simulink library "MCHP_Blockset"  (Simulink 7.5)
(part 3 of 9)

      mask prompts: ACLKCON "Enable fast conversion using Auxiliary clock"; ADC_FRACT "Conversion Format (common to all ADC blocks)"; ADC_NRE "Noise Reduction Enabled (might add delays)"; DMA_Size "Multiple trigger - Vector output - for ADC[0-6] of current block"; ADC_Synchronisation "ADC Sample and Conversion"; ADC_Trig "User defined trigger:"; ADC_TrigTimeStep "Synchronisation with model Time Step:"; ADC_TrigInfo "ADC Trigger Info"; SampleTime "Block output sample time"; ADC_Info "Infos"; ADC0_pin "Analog input pin"; ADC0_R "Input Impedance"; ADC0_res "Resolution of conversion"; ADC0_signed "Output format"; ADC0_FILTER "Filter / Oversampling"; ADC0_FILTER_nSamples "Filter / Oversampling burst of:"; ADC0_STRGEN "Initial trigger option:"; ADC0_STRGEN_on "Initial trigger option:"; ADC0_SSAMPEN "Ensure synchronous sampling (might add a delay)"; ADC0_Info "ADC0 Info"; ADC1_pin "Analog input pin"; ADC1_pin_TXT "ADC0_pin_TXT"; ADC1_R "Input Impedance"; ADC1_res "Resolution of conversion"; ADC1_signed "Output format"; ADC1_FILTER "Filter / Oversampling"; ADC1_FILTER_nSamples "Filter / Oversampling burst of:"; ADC1_STRGEN "Initial trigger option:"; ADC1_STRGEN_on "Initial trigger option:"; ADC1_SSAMPEN "Ensure synchronous sampling (might add a delay)"; ADC1_Info "ADC1 Infos"; ADC2_pin "Analog input pin"; ADC2_R "Input Impedance"; ADC2_res "Resolution of conversion"; ADC2_signed "Output format"; ADC2_FILTER "Filter / Oversampling"; ADC2_FILTER_nSamples "Filter / Oversampling burst of:"; ADC2_STRGEN "Initial trigger option:"; ADC2_STRGEN_on "Initial trigger option:"; ADC2_SSAMPEN "Ensure synchronous sampling (might add a delay)"; ADC2_Info "ADC2 Infos"; ADC3_pin "Analog input pin"; ADC3_R "Input Impedance"; ADC3_res "Resolution of conversion"; ADC3_signed "Output format"; ADC3_FILTER "Filter / Oversampling"; ADC3_FILTER_nSamples "Filter / Oversampling burst of:"; ADC3_STRGEN "Initial trigger option:"; ADC3_STRGEN_on "Initial trigger option:"; ADC3_SSAMPEN "Ensure synchronous sampling (might add a delay)"; ADC3_Info "ADC3 Infos"; ADC4_pin "Analog input pin"; ADC4_R "Input Impedance"; ADC4_res "Resolution of conversion"; ADC4_signed "Output format"; ADC4_FILTER "Filter / Oversampling"; ADC4_FILTER_nSamples "Filter / Oversampling burst of:"; ADC4_STRGEN "Initial trigger option:"; ADC4_STRGEN_on "Initial trigger option:"; ADC4_SSAMPEN "Ensure synchronous sampling (might add a delay)"; ADC4_Info "ADC4 Infos"; ADC5_pin "Analog input pin"; ADC5_R "Input Impedance"; ADC5_res "Resolution of conversion"; ADC5_signed "Output format"; ADC5_FILTER "Filter / Oversampling"; ADC5_FILTER_nSamples "Filter / Oversampling burst of:"; ADC5_STRGEN "Initial trigger option:"; ADC5_STRGEN_on "Initial trigger option:"; ADC5_SSAMPEN "Ensure synchronous sampling (might add a delay)"; ADC5_Info "ADC5 Infos"; ADC6_pin "Analog input pin"; ADC6_R "Input Impedance"; ADC6_res "Resolution of conversion"; ADC6_signed "Output format"; ADC6_FILTER "Filter / Oversampling"; ADC6_FILTER_nSamples "Filter / Oversampling burst of:"; ADC6_STRGEN "Initial trigger option:"; ADC6_STRGEN_on "Initial trigger option:"; ADC6_SSAMPEN "Ensure synchronous sampling (might add a delay)"; ADC6_Info "ADC6 Infos"; ADC7_R "ADC7 Input Impedance (Class 2 and 3 inputs)"; ADC7_res "ADC7 Resolution of conversion (Class 2 and 3 inputs)"; ADC7_AN0 "AN0 pin"; ADC7_AN1 "AN1 pin"; ADC7_AN2 "AN2_pin"; ADC7_AN3 "AN3_pin"; ADC7_AN4 ""; ADC7_AN5 ""; ADC7_AN6 "AN6 / B1 / Pin[32]"; ADC7_AN7 "AN7 / B2 / Pin[33]"; ADC7_AN8 "AN8 / C1 / Pin[31]"; ADC7_AN9 "AN9 / C2 / Pin[36]"; ADC7_AN10 "AN10 / C10 / Pin[28]"; ADC7_AN11 "AN11 / C9 / Pin[27]"; ADC7_AN12 "AN12 / C11 / Pin[19]"; ADC7_AN13 ""; ADC7_AN14 "AN14 / C12 / Pin[20]"; ADC7_AN15 ""; ADC7_AN16 ""; ADC7_AN17 "AN17 / C6 / Pin[4]"; ADC7_AN18 "AN18 / B3 / Pin[34]"; ADC7_AN19 "AN19 / B5 / Pin[43]"; ADC7_AN20 "AN20 / B6 / Pin[44]"; ADC7_AN21 "AN21 / B7 / Pin[1]"; ADC7_AN22 ""; ADC7_AN23 ""; ADC7_AN24 ""; ADC7_AN25 ""; ADC7_AN26 ""; ADC7_AN27 ""; ADC7_AN28 ""; ADC7_AN29 ""; ADC7_AN30 ""; ADC7_AN31 ""; IVref "Vref (1.2V)"; IVTemp "Temp"; ADC7_Info "Shared ADC Infos"
      mask init:
      | MCHP_ADC_HighSpeed_SAR_dsPIC_Callback(gcbh,'INITIALISATION');
      settings: CopyFcn=MCHP_ADC_HighSpeed_SAR_dsPIC_Callback(gcbh,'CopyFcn');  PreSaveFcn=MCHP_Fun.PreSaveFcn_DynamicOptions(gcbh);  OpenFcn=MCHP_ADC_HighSpeed_SAR_dsPIC_Callback(gcbh,'OPEN');
      mask StyleString: popup(Not used|Optimized for PWM resolution & ADC conversion speed|Optimized for PWM accuracy),popup(Integer (right aligned)|Fractional (left aligned)),checkbox,popup(Single trigger - (default)|1 trig / 1 element output (ping pong buffer)|2 trig / 2 elements output (ping-pong buffer)|3 trig / 3 elements output (ping-pong buffer)|4 trig / 4 elements output (ping-pong buffer)),popup(Triggered at end of previous time step|Triggered by custom source|Continuously triggered. Output is last conversion),popup(Dynamic Options),edit,popup(None (independant)|Trig model step after all sample using this trigger are converted|Trig model step after all sample from this block are converted),edit,edit,edit,edit,edit,edit,edit,edit,edit,edit,edit,edit,popup(Dynamic Options),edit,popup(< 200 Ohm|< 500 Ohm|< 1    kOhm|< 2    kOhm|< 5    kOhm|< 10   kOhm|< 20   kOhm|< 50   kOhm|< 100  kOhm|< 200  kOhm|< 500  kOhm|max sampling time),popup(12 bits|10 bits|8 bits|6 bits),popup(unsigned 16 bits|signed 16 bits),popup(No Oversampling|Burst convert of n samples are Summed|Burst convert of n samples are Averaged),popup(2 samples|4 samples|8 samples|16 samples|32 samples|64 samples|128 samples|256 samples),popup(End sampling and start conversion|Start sampling followed by conversion),popup(Start sampling followed by conversion),checkbox,edit,popup(Dynamic Options),edit,popup(< 200 Ohm|< 500 Ohm|< 1    kOhm|< 2    kOhm|< 5    kOhm|< 10   kOhm|< 20   kOhm|< 50   kOhm|< 100  kOhm|< 200  kOhm|< 500  kOhm|max sampling time),popup(12 bits|10 bits|8 bits|6 bits),popup(unsigned 16 bits|signed 16 bits),popup(No Oversampling|Burst convert of n samples are Summed|Burst convert of n samples are Averaged),popup(2 samples|4 samples|8 samples|16 samples|32 samples|64 samples|128 samples|256 samples),popup(End sampling and start conversion|Start sampling followed by conversion),popup(Start sampling followed by conversion),checkbox,edit,popup(Dynamic Options),edit,popup(< 200 Ohm|< 500 Ohm|< 1    kOhm|< 2    kOhm|< 5    kOhm|< 10   kOhm|< 20   kOhm|< 50   kOhm|< 100  kOhm|< 200  kOhm|< 500  kOhm|max sampling time),popup(12 bits|10 bits|8 bits|6 bits),popup(unsigned 16 bits|signed 16 bits),popup(No Oversampling|Burst convert of n samples are Summed|Burst convert of n samples are Averaged),popup(2 samples|4 samples|8 samples|16 samples|32 samples|64 samples|128 samples|256 samples),popup(End sampling and start conversion|Start sampling followed by conversion),popup(Start sampling followed by conversion),checkbox,edit,popup(Dynamic Options),edit,popup(< 200 Ohm|< 500 Ohm|< 1    kOhm|< 2    kOhm|< 5    kOhm|< 10   kOhm|< 20   kOhm|< 50   kOhm|< 100  kOhm|< 200  kOhm|< 500  kOhm|max sampling time),popup(12 bits|10 bits|8 bits|6 bits),popup(unsigned 16 bits|signed 16 bits),popup(No Oversampling|Burst convert of n samples are Summed|Burst convert of n samples are Averaged),popup(2 samples|4 samples|8 samples|16 samples|32 samples|64 samples|128 samples|256 samples),popup(End sampling and start conversion|Start sampling followed by conversion),popup(Start sampling followed by conversion),checkbox,edit,popup(Dynamic Options),edit,popup(< 200 Ohm|< 500 Ohm|< 1    kOhm|< 2    kOhm|< 5    kOhm|< 10   kOhm|< 20   kOhm|< 50   kOhm|< 100  kOhm|< 200  kOhm|< 500  kOhm|max sampling time),popup(12 bits|10 bits|8 bits|6 bits),popup(unsigned 16 bits|signed 16 bits),popup(No Oversampling|Burst convert of n samples are Summed|Burst convert of n samples are Averaged),popup(2 samples|4 samples|8 samples|16 samples|32 samples|64 samples|128 samples|256 samples),popup(End sampling and start conversion|Start sampling followed by conversion),popup(Start sampling followed by conversion),checkbox,edit,popup(Dynamic Options),edit,popup(< 200 Ohm|< 500 Ohm|< 1    kOhm|< 2    kOhm|< 5    kOhm|< 10   kOhm|< 20   kOhm|< 50   kOhm|< 100  kOhm|< 200  kOhm|< 500  kOhm|max sampling time),popup(12 bits|10 bits|8 bits|6 bits),popup(unsigned 16 bits|signed 16 bits),popup(No Oversampling|Burst convert of n samples are Summed|Burst convert of n samples are Averaged),popup(2 samples|4 samples|8 samples|16 samples|32 samples|64 samples|128 samples|256 samples),popup(End sampling and start conversion|Start sampling followed by conversion),popup(Start sampling followed by conversion),checkbox,edit,popup(Dynamic Options),edit,popup(< 200 Ohm|< 500 Ohm|< 1    kOhm|< 2    kOhm|< 5    kOhm|< 10   kOhm|< 20   kOhm|< 50   kOhm|< 100  kOhm|< 200  kOhm|< 500  kOhm|max sampling time),popup(12 bits|10 bits|8 bits|6 bits),popup(unsigned 16 bits|signed 16 bits),popup(No Oversampling|Burst convert of n samples are Summed|Burst convert of n samples are Averaged),popup(2 samples|4 samples|8 samples|16 samples|32 samples|64 samples|128 samples|256 samples),popup(End sampling and start conversion|Start sampling followed by conversion),popup(Start sampling followed by conversion),checkbox,edit,popup(< 200 Ohm|< 500 Ohm|< 1    kOhm|< 2    kOhm|< 5    kOhm|< 10   kOhm|< 20   kOhm|< 50   kOhm|< 100  kOhm|< 200  kOhm|< 500  kOhm|max sampling time),popup(12 bits|10 bits|8 bits|6 bits),popup(Not used|unsigned int16 |signed int16|---Burst Sample with internal Digital filter---|2 samples averaged - unsigned int16|4 samples averaged - unsigned int16|8 samples averaged - unsigned int16|16 samples averaged - unsigned int16|32 samples averaged - unsigned int16|64 samples averaged - unsigned int16|128 samples averaged - unsigned int16|256 samples averaged - unsigned int16|----|2 samples averaged - signed int16|4 samples averaged - signed int16|8 samples averaged - signed int16|16 samples averaged - signed int16|32 samples averaged - signed int16|64 samples averaged - signed int16|128 samples averaged - signed int16|256 samples averaged - signed int16|-----|4 samples summed - unsigned int16|8 samples summed - unsigned int16|16 samples summed - unsigned int16|32 samples summed - unsigned int16|64 samples summed - unsigned int16|128 samples summed - unsigned int16|256 samples summed - unsigned int16|------|2 samples summed - signed int16|4 samples summed - signed int16|8 samples summed - signed int16|16 samples summed - signed int16|32 samples summed - signed int16),popup(Not used|unsigned int16 |signed int16|---Burst Sample with internal Digital filter---|2 samples averaged - unsigned int16|4 samples averaged - unsigned int16|8 samples averaged - unsigned int16|16 samples averaged - unsigned int16|32 samples averaged - unsigned int16|64 samples averaged - unsigned int16|128 samples averaged - unsigned int16|256 samples averaged - unsigned int16|----|2 samples averaged - signed int16|4 samples averaged - signed int16|8 samples averaged - signed int16|16 samples averaged - signed int16|32 samples averaged - signed int16|64 samples averaged - signed int16|128 samples averaged - signed int16|256 samples averaged - signed int16|-----|4 samples summed - unsigned int16|8 samples summed - unsigned int16|16 samples summed - unsigned int16|32 samples summed - unsigned int16|64 samples summed - unsigned int16|128 samples summed - unsigned int16|256 samples summed - unsigned int16|------|2 samples summed - signed int16|4 samples summed - signed int16|8 samples summed - signed int16|16 samples summed - signed int16|32 samples summed - signed int16|64 samples summed - signed int16|128 samples summed - signed int16|256 samples summed - signed int16),popup(Not used|unsigned int16 |signed int16|---Burst Sample with internal Digital filter---|2 samples averaged - unsigned int16|4 samples averaged - unsigned int16|8 samples averaged - unsigned int16|16 samples averaged - unsigned int16|32 samples averaged - unsigned int16|64 samples averaged - unsigned int16|128 samples averaged - unsigned int16|256 samples averaged - unsigned int16|----|2 samples averaged - signed int16|4 samples averaged - signed int16|8 samples averaged - signed int16|16 samples averaged - signed int16|32 samples averaged - signed int16|64 samples averaged - signed int16|128 samples averaged - signed int16|256 samples averaged - signed int16|-----|4 samples summed - unsigned int16|8 samples summed - unsigned int16|16 samples summed - unsigned int16|32 samples summed - unsigned int16|64 samples summed - unsigned int16|128 samples summed - unsigned int16|256 samples summed - unsigned int16|------|2 samples summed - signed int16|4 samples summed - signed int16|8 samples summed - signed int16|16 samples summed - signed int16|32 samples summed - signed int16|64 samples summed - signed int16|128 samples summed - signed int16|256 samples summed - signed int16),popup(Not used|unsigned int16 |signed int16|---Burst Sample with internal Digital filter---|2 samples averaged - unsigned int16|4 samples averaged - unsigned int16|8 samples averaged - unsigned int16|16 samples averaged - unsigned int16|32 samples averaged - unsigned int16|64 samples averaged - unsigned int16|128 samples averaged - unsigned int16|256 samples averaged - unsigned int16|----|2 samples averaged - signed int16|4 samples averaged - signed int16|8 samples averaged - signed int16|16 samples averaged - signed int16|32 samples averaged - signed int16|64 samples averaged - signed int16|128 samples averaged - signed int16|256 samples averaged - signed int16|-----|4 samples summed - unsigned int16|8 samples summed - unsigned int16|16 samples summed - unsigned int16|32 samples summed - unsigned int16|64 samples summed - unsigned int16|128 samples summed - unsigned int16|256 samples summed - unsigned int16|------|2 samples summed - signed int16|4 samples summed - signed int16|8 samples summed - signed int16|16 samples summed - signed int16|32 samples summed - signed int16|64 samples summed - signed int16|128 samples summed - signed int16|256 samples summed - signed int16),popup(Not used|unsigned int16 |signed int16|---Burst Sample with internal Digital filter---|2 samples averaged - unsigned int16|4 samples averaged - unsigned int16|8 samples averaged - unsigned int16|16 samples averaged - unsigned int16|32 samples averaged - unsigned int16|64 samples averaged - unsigned int16|128 samples averaged - unsigned int16|256 samples averaged - unsigned int16|----|2 samples averaged - signed int16|4 samples averaged - signed int16|8 samples averaged - signed int16|16 samples averaged - signed int16|32 samples averaged - signed int16|64 samples averaged - signed int16|128 samples averaged - signed int16|256 samples averaged - signed int16|-----|4 samples summed - unsigned int16|8 samples summed - unsigned int16|16 samples summed - unsigned int16|32 samples summed - unsigned int16|64 samples summed - unsigned int16|128 samples summed - unsigned int16|256 samples summed - unsigned int16|------|2 samples summed - signed int16|4 samples summed - signed int16|8 samples summed - signed int16|16 samples summed - signed int16|32 samples summed - signed int16|64 samples summed - signed int16|128 samples summed - signed int16|256 samples summed - signed int16),popup(Not used|unsigned int16 |signed int16|---Burst Sample with internal Digital filter---|2 samples averaged - unsigned int16|4 samples averaged - unsigned int16|8 samples averaged - unsigned int16|16 samples averaged - unsigned int16|32 samples averaged - unsigned int16|64 samples averaged - unsigned int16|128 samples averaged - unsigned int16|256 samples averaged - unsigned int16|----|2 samples averaged - signed int16|4 samples averaged - signed int16|8 samples averaged - signed int16|16 samples averaged - signed int16|32 samples averaged - signed int16|64 samples averaged - signed int16|128 samples averaged - signed int16|256 samples averaged - signed int16|-----|4 samples summed - unsigned int16|8 samples summed - unsigned int16|16 samples summed - unsigned int16|32 samples summed - unsigned int16|64 samples summed - unsigned int16|128 samples summed - unsigned int16|256 samples summed - unsigned int16|------|2 samples summed - signed int16|4 samples summed - signed int16|8 samples summed - signed int16|16 samples summed - signed int16|32 samples summed - signed int16|64 samples summed - signed int16|128 samples summed - signed int16|256 samples summed - signed int16),popup(Not used|unsigned int16 |signed int16|---Burst Sample with internal Digital filter---|2 samples averaged - unsigned int16|4 samples averaged - unsigned int16|8 samples averaged - unsigned int16|16 samples averaged - unsigned int16|32 samples averaged - unsigned int16|64 samples averaged - unsigned int16|128 samples averaged - unsigned int16|256 samples averaged - unsigned int16|----|2 samples averaged - signed int16|4 samples averaged - signed int16|8 samples averaged - signed int16|16 samples averaged - signed int16|32 samples averaged - signed int16|64 samples averaged - signed int16|128 samples averaged - signed int16|256 samples averaged - signed int16|-----|4 samples summed - unsigned int16|8 samples summed - unsigned int16|16 samples summed - unsigned int16|32 samples summed - unsigned int16|64 samples summed - unsigned int16|128 samples summed - unsigned int16|256 samples summed - unsigned int16|------|2 samples summed - signed int16|4 samples summed - signed int16|8 samples summed - signed int16|16 samples summed - signed int16|32 samples summed - signed int16|64 samples summed - signed int16|128 samples summed - signed int16|256 samples summed - signed int16),popup(Not used|unsigned int16 |signed int16|---Burst Sample with internal Digital filter---|2 samples averaged - unsigned int16|4 samples averaged - unsigned int16|8 samples averaged - unsigned int16|16 samples averaged - unsigned int16|32 samples averaged - unsigned int16|64 samples averaged - unsigned int16|128 samples averaged - unsigned int16|256 samples averaged - unsigned int16|----|2 samples averaged - signed int16|4 samples averaged - signed int16|8 samples averaged - signed int16|16 samples averaged - signed int16|32 samples averaged - signed int16|64 samples averaged - signed int16|128 samples averaged - signed int16|256 samples averaged - signed int16|-----|4 samples summed - unsigned int16|8 samples summed - unsigned int16|16 samples summed - unsigned int16|32 samples summed - unsigned int16|64 samples summed - unsigned int16|128 samples summed - unsigned int16|256 samples summed - unsigned int16|------|2 samples summed - signed int16|4 samples summed - signed int16|8 samples summed - signed int16|16 samples summed - signed int16|32 samples summed - signed int16|64 samples summed - signed int16|128 samples summed - signed int16|256 samples summed - signed int16),popup(Not used|unsigned int16 |signed int16|---Burst Sample with internal Digital filter---|2 samples averaged - unsigned int16|4 samples averaged - unsigned int16|8 samples averaged - unsigned int16|16 samples averaged - unsigned int16|32 samples averaged - unsigned int16|64 samples averaged - unsigned int16|128 samples averaged - unsigned int16|256 samples averaged - unsigned int16|----|2 samples averaged - signed int16|4 samples averaged - signed int16|8 samples averaged - signed int16|16 samples averaged - signed int16|32 samples averaged - signed int16|64 samples averaged - signed int16|128 samples averaged - signed int16|256 samples averaged - signed int16|-----|4 samples summed - unsigned int16|8 samples summed - unsigned int16|16 samples summed - unsigned int16|32 samples summed - unsigned int16|64 samples summed - unsigned int16|128 samples summed - unsigned int16|256 samples summed - unsigned int16|------|2 samples summed - signed int16|4 samples summed - signed int16|8 samples summed - signed int16|16 samples summed - signed int16|32 samples summed - signed int16|64 samples summed - signed int16|128 samples summed - signed int16|256 samples summed - signed int16),popup(Not used|unsigned int16 |signed int16|---Burst Sample with internal Digital filter---|2 samples averaged - unsigned int16|4 samples averaged - unsigned int16|8 samples averaged - unsigned int16|16 samples averaged - unsigned int16|32 samples averaged - unsigned int16|64 samples averaged - unsigned int16|128 samples averaged - unsigned int16|256 samples averaged - unsigned int16|----|2 samples averaged - signed int16|4 samples averaged - signed int16|8 samples averaged - signed int16|16 samples averaged - signed int16|32 samples averaged - signed int16|64 samples averaged - signed int16|128 samples averaged - signed int16|256 samples averaged - signed int16|-----|4 samples summed - unsigned int16|8 samples summed - unsigned int16|16 samples summed - unsigned int16|32 samples summed - unsigned int16|64 samples summed - unsigned int16|128 samples summed - unsigned int16|256 samples summed - unsigned int16|------|2 samples summed - signed int16|4 samples summed - signed int16|8 samples summed - signed int16|16 samples summed - signed int16|32 samples summed - signed int16|64 samples summed - signed int16|128 samples summed - signed int16|256 samples summed - signed int16),popup(Not used|unsigned int16 |signed int16|---Burst Sample with internal Digital filter---|2 samples averaged - unsigned int16|4 samples averaged - unsigned int16|8 samples averaged - unsigned int16|16 samples averaged - unsigned int16|32 samples averaged - unsigned int16|64 samples averaged - unsigned int16|128 samples averaged - unsigned int16|256 samples averaged - unsigned int16|----|2 samples averaged - signed int16|4 samples averaged - signed int16|8 samples averaged - signed int16|16 samples averaged - signed int16|32 samples averaged - signed int16|64 samples averaged - signed int16|128 samples averaged - signed int16|256 samples averaged - signed int16|-----|4 samples summed - unsigned int16|8 samples summed - unsigned int16|16 samples summed - unsigned int16|32 samples summed - unsigned int16|64 samples summed - unsigned int16|128 samples summed - unsigned int16|256 samples summed - unsigned int16|------|2 samples summed - signed int16|4 samples summed - signed int16|8 samples summed - signed int16|16 samples summed - signed int16|32 samples summed - signed int16|64 samples summed - signed int16|128 samples summed - signed int16|256 samples summed - signed int16),popup(Not used|unsigned int16 |signed int16|---Burst Sample with internal Digital filter---|2 samples averaged - unsigned int16|4 samples averaged - unsigned int16|8 samples averaged - unsigned int16|16 samples averaged - unsigned int16|32 samples averaged - unsigned int16|64 samples averaged - unsigned int16|128 samples averaged - unsigned int16|256 samples averaged - unsigned int16|----|2 samples averaged - signed int16|4 samples averaged - signed int16|8 samples averaged - signed int16|16 samples averaged - signed int16|32 samples averaged - signed int16|64 samples averaged - signed int16|128 samples averaged - signed int16|256 samples averaged - signed int16|-----|4 samples summed - unsigned int16|8 samples summed - unsigned int16|16 samples summed - unsigned int16|32 samples summed - unsigned int16|64 samples summed - unsigned int16|128 samples summed - unsigned int16|256 samples summed - unsigned int16|------|2 samples summed - signed int16|4 samples summed - signed int16|8 samples summed - signed int16|16 samples summed - signed int16|32 samples summed - signed int16|64 samples summed - signed int16|128 samples summed - signed int16|256 samples summed - signed int16),popup(Not used|unsigned int16 |signed int16|---Burst Sample with internal Digital filter---|2 samples averaged - unsigned int16|4 samples averaged - unsigned int16|8 samples averaged - unsigned int16|16 samples averaged - unsigned int16|32 samples averaged - unsigned int16|64 samples averaged - unsigned int16|128 samples averaged - unsigned int16|256 samples averaged - unsigned int16|----|2 samples averaged - signed int16|4 samples averaged - signed int16|8 samples averaged - signed int16|16 samples averaged - signed int16|32 samples averaged - signed int16|64 samples averaged - signed int16|128 samples averaged - signed int16|256 samples averaged - signed int16|-----|4 samples summed - unsigned int16|8 samples summed - unsigned int16|16 samples summed - unsigned int16|32 samples summed - unsigned int16|64 samples summed - unsigned int16|128 samples summed - unsigned int16|256 samples summed - unsigned int16|------|2 samples summed - signed int16|4 samples summed - signed int16|8 samples summed - signed int16|16 samples summed - signed int16|32 samples summed - signed int16|64 samples summed - signed int16|128 samples summed - signed int16|256 samples summed - signed int16),popup(Not used|unsigned int16 |signed int16|---Burst Sample with internal Digital filter---|2 samples averaged - unsigned int16|4 samples averaged - unsigned int16|8 samples averaged - unsigned int16|16 samples averaged - unsigned int16|32 samples averaged - unsigned int16|64 samples averaged - unsigned int16|128 samples averaged - unsigned int16|256 samples averaged - unsigned int16|----|2 samples averaged - signed int16|4 samples averaged - signed int16|8 samples averaged - signed int16|16 samples averaged - signed int16|32 samples averaged - signed int16|64 samples averaged - signed int16|128 samples averaged - signed int16|256 samples averaged - signed int16|-----|4 samples summed - unsigned int16|8 samples summed - unsigned int16|16 samples summed - unsigned int16|32 samples summed - unsigned int16|64 samples summed - unsigned int16|128 samples summed - unsigned int16|256 samples summed - unsigned int16|------|2 samples summed - signed int16|4 samples summed - signed int16|8 samples summed - signed int16|16 samples summed - signed int16|32 samples summed - signed int16|64 samples summed - signed int16|128 samples summed - signed int16|256 samples summed - signed int16),popup(Not used|unsigned int16 |signed int16|---Burst Sample with internal Digital filter---|2 samples averaged - unsigned int16|4 samples averaged - unsigned int16|8 samples averaged - unsigned int16|16 samples averaged - unsigned int16|32 samples averaged - unsigned int16|64 samples averaged - unsigned int16|128 samples averaged - unsigned int16|256 samples averaged - unsigned int16|----|2 samples averaged - signed int16|4 samples averaged - signed int16|8 samples averaged - signed int16|16 samples averaged - signed int16|32 samples averaged - signed int16|64 samples averaged - signed int16|128 samples averaged - signed int16|256 samples averaged - signed int16|-----|4 samples summed - unsigned int16|8 samples summed - unsigned int16|16 samples summed - unsigned int16|32 samples summed - unsigned int16|64 samples summed - unsigned int16|128 samples summed - unsigned int16|256 samples summed - unsigned int16|------|2 samples summed - signed int16|4 samples summed - signed int16|8 samples summed - signed int16|16 samples summed - signed int16|32 samples summed - signed int16|64 samples summed - signed int16|128 samples summed - signed int16|256 samples summed - signed int16),popup(Not used|unsigned int16 |signed int16|---Burst Sample with internal Digital filter---|2 samples averaged - unsigned int16|4 samples averaged - unsigned int16|8 samples averaged - unsigned int16|16 samples averaged - unsigned int16|32 samples averaged - unsigned int16|64 samples averaged - unsigned int16|128 samples averaged - unsigned int16|256 samples averaged - unsigned int16|----|2 samples averaged - signed int16|4 samples averaged - signed int16|8 samples averaged - signed int16|16 samples averaged - signed int16|32 samples averaged - signed int16|64 samples averaged - signed int16|128 samples averaged - signed int16|256 samples averaged - signed int16|-----|4 samples summed - unsigned int16|8 samples summed - unsigned int16|16 samples summed - unsigned int16|32 samples summed - unsigned int16|64 samples summed - unsigned int16|128 samples summed - unsigned int16|256 samples summed - unsigned int16|------|2 samples summed - signed int16|4 samples summed - signed int16|8 samples summed - signed int16|16 samples summed - signed int16|32 samples summed - signed int16|64 samples summed - signed int16|128 samples summed - signed int16|256 samples summed - signed int16),popup(Not used|unsigned int16 |signed int16|---Burst Sample with internal Digital filter---|2 samples averaged - unsigned int16|4 samples averaged - unsigned int16|8 samples averaged - unsigned int16|16 samples averaged - unsigned int16|32 samples averaged - unsigned int16|64 samples averaged - unsigned int16|128 samples averaged - unsigned int16|256 samples averaged - unsigned int16|----|2 samples averaged - signed int16|4 samples averaged - signed int16|8 samples averaged - signed int16|16 samples averaged - signed int16|32 samples averaged - signed int16|64 samples averaged - signed int16|128 samples averaged - signed int16|256 samples averaged - signed int16|-----|4 samples summed - unsigned int16|8 samples summed - unsigned int16|16 samples summed - unsigned int16|32 samples summed - unsigned int16|64 samples summed - unsigned int16|128 samples summed - unsigned int16|256 samples summed - unsigned int16|------|2 samples summed - signed int16|4 samples summed - signed int16|8 samples summed - signed int16|16 samples summed - signed int16|32 samples summed - signed int16|64 samples summed - signed int16|128 samples summed - signed int16|256 samples summed - signed int16),popup(Not used|unsigned int16 |signed int16|---Burst Sample with internal Digital filter---|2 samples averaged - unsigned int16|4 samples averaged - unsigned int16|8 samples averaged - unsigned int16|16 samples averaged - unsigned int16|32 samples averaged - unsigned int16|64 samples averaged - unsigned int16|128 samples averaged - unsigned int16|256 samples averaged - unsigned int16|----|2 samples averaged - signed int16|4 samples averaged - signed int16|8 samples averaged - signed int16|16 samples averaged - signed int16|32 samples averaged - signed int16|64 samples averaged - signed int16|128 samples averaged - signed int16|256 samples averaged - signed int16|-----|4 samples summed - unsigned int16|8 samples summed - unsigned int16|16 samples summed - unsigned int16|32 samples summed - unsigned int16|64 samples summed - unsigned int16|128 samples summed - unsigned int16|256 samples summed - unsigned int16|------|2 samples summed - signed int16|4 samples summed - signed int16|8 samples summed - signed int16|16 samples summed - signed int16|32 samples summed - signed int16|64 samples summed - signed int16|128 samples summed - signed int16|256 samples summed - signed int16),popup(Not used|unsigned int16 |signed int16|---Burst Sample with internal Digital filter---|2 samples averaged - unsigned int16|4 samples averaged - unsigned int16|8 samples averaged - unsigned int16|16 samples averaged - unsigned int16|32 samples averaged - unsigned int16|64 samples averaged - unsigned int16|128 samples averaged - unsigned int16|256 samples averaged - unsigned int16|----|2 samples averaged - signed int16|4 samples averaged - signed int16|8 samples averaged - signed int16|16 samples averaged - signed int16|32 samples averaged - signed int16|64 samples averaged - signed int16|128 samples averaged - signed int16|256 samples averaged - signed int16|-----|4 samples summed - unsigned int16|8 samples summed - unsigned int16|16 samples summed - unsigned int16|32 samples summed - unsigned int16|64 samples summed - unsigned int16|128 samples summed - unsigned int16|256 samples summed - unsigned int16|------|2 samples summed - signed int16|4 samples summed - signed int16|8 samples summed - signed int16|16 samples summed - signed int16|32 samples summed - signed int16|64 samples summed - signed int16|128 samples summed - signed int16|256 samples summed - signed int16),popup(Not used|unsigned int16 |signed int16|---Burst Sample with internal Digital filter---|2 samples averaged - unsigned int16|4 samples averaged - unsigned int16|8 samples averaged - unsigned int16|16 samples averaged - unsigned int16|32 samples averaged - unsigned int16|64 samples averaged - unsigned int16|128 samples averaged - unsigned int16|256 samples averaged - unsigned int16|----|2 samples averaged - signed int16|4 samples averaged - signed int16|8 samples averaged - signed int16|16 samples averaged - signed int16|32 samples averaged - signed int16|64 samples averaged - signed int16|128 samples averaged - signed int16|256 samples averaged - signed int16|-----|4 samples summed - unsigned int16|8 samples summed - unsigned int16|16 samples summed - unsigned int16|32 samples summed - unsigned int16|64 samples summed - unsigned int16|128 samples summed - unsigned int16|256 samples summed - unsigned int16|------|2 samples summed - signed int16|4 samples summed - signed int16|8 samples summed - signed int16|16 samples summed - signed int16|32 samples summed - signed int16|64 samples summed - signed int16|128 samples summed - signed int16|256 samples summed - signed int16),popup(Not used|unsigned int16 |signed int16|---Burst Sample with internal Digital filter---|2 samples averaged - unsigned int16|4 samples averaged - unsigned int16|8 samples averaged - unsigned int16|16 samples averaged - unsigned int16|32 samples averaged - unsigned int16|64 samples averaged - unsigned int16|128 samples averaged - unsigned int16|256 samples averaged - unsigned int16|----|2 samples averaged - signed int16|4 samples averaged - signed int16|8 samples averaged - signed int16|16 samples averaged - signed int16|32 samples averaged - signed int16|64 samples averaged - signed int16|128 samples averaged - signed int16|256 samples averaged - signed int16|-----|4 samples summed - unsigned int16|8 samples summed - unsigned int16|16 samples summed - unsigned int16|32 samples summed - unsigned int16|64 samples summed - unsigned int16|128 samples summed - unsigned int16|256 samples summed - unsigned int16|------|2 samples summed - signed int16|4 samples summed - signed int16|8 samples summed - signed int16|16 samples summed - signed int16|32 samples summed - signed int16|64 samples summed - signed int16|128 samples summed - signed int16|256 samples summed - signed int16),popup(Not used|unsigned int16 |signed int16|---Burst Sample with internal Digital filter---|2 samples averaged - unsigned int16|4 samples averaged - unsigned int16|8 samples averaged - unsigned int16|16 samples averaged - unsigned int16|32 samples averaged - unsigned int16|64 samples averaged - unsigned int16|128 samples averaged - unsigned int16|256 samples averaged - unsigned int16|----|2 samples averaged - signed int16|4 samples averaged - signed int16|8 samples averaged - signed int16|16 samples averaged - signed int16|32 samples averaged - signed int16|64 samples averaged - signed int16|128 samples averaged - signed int16|256 samples averaged - signed int16|-----|4 samples summed - unsigned int16|8 samples summed - unsigned int16|16 samples summed - unsigned int16|32 samples summed - unsigned int16|64 samples summed - unsigned int16|128 samples summed - unsigned int16|256 samples summed - unsigned int16|------|2 samples summed - signed int16|4 samples summed - signed int16|8 samples summed - signed int16|16 samples summed - signed int16|32 samples summed - signed int16|64 samples summed - signed int16|128 samples summed - signed int16|256 samples summed - signed int16),popup(Not used|unsigned int16 |signed int16|---Burst Sample with internal Digital filter---|2 samples averaged - unsigned int16|4 samples averaged - unsigned int16|8 samples averaged - unsigned int16|16 samples averaged - unsigned int16|32 samples averaged - unsigned int16|64 samples averaged - unsigned int16|128 samples averaged - unsigned int16|256 samples averaged - unsigned int16|----|2 samples averaged - signed int16|4 samples averaged - signed int16|8 samples averaged - signed int16|16 samples averaged - signed int16|32 samples averaged - signed int16|64 samples averaged - signed int16|128 samples averaged - signed int16|256 samples averaged - signed int16|-----|4 samples summed - unsigned int16|8 samples summed - unsigned int16|16 samples summed - unsigned int16|32 samples summed - unsigned int16|64 samples summed - unsigned int16|128 samples summed - unsigned int16|256 samples summed - unsigned int16|------|2 samples summed - signed int16|4 samples summed - signed int16|8 samples summed - signed int16|16 samples summed - signed int16|32 samples summed - signed int16|64 samples summed - signed int16|128 samples summed - signed int16|256 samples summed - signed int16),popup(Not used|unsigned int16 |signed int16|---Burst Sample with internal Digital filter---|2 samples averaged - unsigned int16|4 samples averaged - unsigned int16|8 samples averaged - unsigned int16|16 samples averaged - unsigned int16|32 samples averaged - unsigned int16|64 samples averaged - unsigned int16|128 samples averaged - unsigned int16|256 samples averaged - unsigned int16|----|2 samples averaged - signed int16|4 samples averaged - signed int16|8 samples averaged - signed int16|16 samples averaged - signed int16|32 samples averaged - signed int16|64 samples averaged - signed int16|128 samples averaged - signed int16|256 samples averaged - signed int16|-----|4 samples summed - unsigned int16|8 samples summed - unsigned int16|16 samples summed - unsigned int16|32 samples summed - unsigned int16|64 samples summed - unsigned int16|128 samples summed - unsigned int16|256 samples summed - unsigned int16|------|2 samples summed - signed int16|4 samples summed - signed int16|8 samples summed - signed int16|16 samples summed - signed int16|32 samples summed - signed int16|64 samples summed - signed int16|128 samples summed - signed int16|256 samples summed - signed int16),popup(Not used|unsigned int16 |signed int16|---Burst Sample with internal Digital filter---|2 samples averaged - unsigned int16|4 samples averaged - unsigned int16|8 samples averaged - unsigned int16|16 samples averaged - unsigned int16|32 samples averaged - unsigned int16|64 samples averaged - unsigned int16|128 samples averaged - unsigned int16|256 samples averaged - unsigned int16|----|2 samples averaged - signed int16|4 samples averaged - signed int16|8 samples averaged - signed int16|16 samples averaged - signed int16|32 samples averaged - signed int16|64 samples averaged - signed int16|128 samples averaged - signed int16|256 samples averaged - signed int16|-----|4 samples summed - unsigned int16|8 samples summed - unsigned int16|16 samples summed - unsigned int16|32 samples summed - unsigned int16|64 samples summed - unsigned int16|128 samples summed - unsigned int16|256 samples summed - unsigned int16|------|2 samples summed - signed int16|4 samples summed - signed int16|8 samples summed - signed int16|16 samples summed - signed int16|32 samples summed - signed int16|64 samples summed - signed int16|128 samples summed - signed int16|256 samples summed - signed int16),popup(Not used|unsigned int16 |signed int16|---Burst Sample with internal Digital filter---|2 samples averaged - unsigned int16|4 samples averaged - unsigned int16|8 samples averaged - unsigned int16|16 samples averaged - unsigned int16|32 samples averaged - unsigned int16|64 samples averaged - unsigned int16|128 samples averaged - unsigned int16|256 samples averaged - unsigned int16|----|2 samples averaged - signed int16|4 samples averaged - signed int16|8 samples averaged - signed int16|16 samples averaged - signed int16|32 samples averaged - signed int16|64 samples averaged - signed int16|128 samples averaged - signed int16|256 samples averaged - signed int16|-----|4 samples summed - unsigned int16|8 samples summed - unsigned int16|16 samples summed - unsigned int16|32 samples summed - unsigned int16|64 samples summed - unsigned int16|128 samples summed - unsigned int16|256 samples summed - unsigned int16|------|2 samples summed - signed int16|4 samples summed - signed int16|8 samples summed - signed int16|16 samples summed - signed int16|32 samples summed - signed int16|64 samples summed - signed int16|128 samples summed - signed int16|256 samples summed - signed int16),popup(Not used|unsigned int16 |signed int16|---Burst Sample with internal Digital filter---|2 samples averaged - unsigned int16|4 samples averaged - unsigned int16|8 samples averaged - unsigned int16|16 samples averaged - unsigned int16|32 samples averaged - unsigned int16|64 samples averaged - unsigned int16|128 samples averaged - unsigned int16|256 samples averaged - unsigned int16|----|2 samples averaged - signed int16|4 samples averaged - signed int16|8 samples averaged - signed int16|16 samples averaged - signed int16|32 samples averaged - signed int16|64 samples averaged - signed int16|128 samples averaged - signed int16|256 samples averaged - signed int16|-----|4 samples summed - unsigned int16|8 samples summed - unsigned int16|16 samples summed - unsigned int16|32 samples summed - unsigned int16|64 samples summed - unsigned int16|128 samples summed - unsigned int16|256 samples summed - unsigned int16|------|2 samples summed - signed int16|4 samples summed - signed int16|8 samples summed - signed int16|16 samples summed - signed int16|32 samples summed - signed int16|64 samples summed - signed int16|128 samples summed - signed int16|256 samples summed - signed int16),popup(Not used|unsigned int16 |signed int16|---Burst Sample with internal Digital filter---|2 samples averaged - unsigned int16|4 samples averaged - unsigned int16|8 samples averaged - unsigned int16|16 samples averaged - unsigned int16|32 samples averaged - unsigned int16|64 samples averaged - unsigned int16|128 samples averaged - unsigned int16|256 samples averaged - unsigned int16|----|2 samples averaged - signed int16|4 samples averaged - signed int16|8 samples averaged - signed int16|16 samples averaged - signed int16|32 samples averaged - signed int16|64 samples averaged - signed int16|128 samples averaged - signed int16|256 samples averaged - signed int16|-----|4 samples summed - unsigned int16|8 samples summed - unsigned int16|16 samples summed - unsigned int16|32 samples summed - unsigned int16|64 samples summed - unsigned int16|128 samples summed - unsigned int16|256 samples summed - unsigned int16|------|2 samples summed - signed int16|4 samples summed - signed int16|8 samples summed - signed int16|16 samples summed - signed int16|32 samples summed - signed int16|64 samples summed - signed int16|128 samples summed - signed int16|256 samples summed - signed int16),popup(Not used|unsigned int16 |signed int16|---Burst Sample with internal Digital filter---|2 samples averaged - unsigned int16|4 samples averaged - unsigned int16|8 samples averaged - unsigned int16|16 samples averaged - unsigned int16|32 samples averaged - unsigned int16|64 samples averaged - unsigned int16|128 samples averaged - unsigned int16|256 samples averaged - unsigned int16|----|2 samples averaged - signed int16|4 samples averaged - signed int16|8 samples averaged - signed int16|16 samples averaged - signed int16|32 samples averaged - signed int16|64 samples averaged - signed int16|128 samples averaged - signed int16|256 samples averaged - signed int16|-----|4 samples summed - unsigned int16|8 samples summed - unsigned int16|16 samples summed - unsigned int16|32 samples summed - unsigned int16|64 samples summed - unsigned int16|128 samples summed - unsigned int16|256 samples summed - unsigned int16|------|2 samples summed - signed int16|4 samples summed - signed int16|8 samples summed - signed int16|16 samples summed - signed int16|32 samples summed - signed int16|64 samples summed - signed int16|128 samples summed - signed int16|256 samples summed - signed int16),popup(Not used|unsigned int16 |signed int16|---Burst Sample with internal Digital filter---|2 samples averaged - unsigned int16|4 samples averaged - unsigned int16|8 samples averaged - unsigned int16|16 samples averaged - unsigned int16|32 samples averaged - unsigned int16|64 samples averaged - unsigned int16|128 samples averaged - unsigned int16|256 samples averaged - unsigned int16|----|2 samples averaged - signed int16|4 samples averaged - signed int16|8 samples averaged - signed int16|16 samples averaged - signed int16|32 samples averaged - signed int16|64 samples averaged - signed int16|128 samples averaged - signed int16|256 samples averaged - signed int16|-----|4 samples summed - unsigned int16|8 samples summed - unsigned int16|16 samples summed - unsigned int16|32 samples summed - unsigned int16|64 samples summed - unsigned int16|128 samples summed - unsigned int16|256 samples summed - unsigned int16|------|2 samples summed - signed int16|4 samples summed - signed int16|8 samples summed - signed int16|16 samples summed - signed int16|32 samples summed - signed int16|64 samples summed - signed int16|128 samples summed - signed int16|256 samples summed - signed int16),popup(Not used|unsigned int16 |signed int16|---Burst Sample with internal Digital filter---|2 samples averaged - unsigned int16|4 samples averaged - unsigned int16|8 samples averaged - unsigned int16|16 samples averaged - unsigned int16|32 samples averaged - unsigned int16|64 samples averaged - unsigned int16|128 samples averaged - unsigned int16|256 samples averaged - unsigned int16|----|2 samples averaged - signed int16|4 samples averaged - signed int16|8 samples averaged - signed int16|16 samples averaged - signed int16|32 samples averaged - signed int16|64 samples averaged - signed int16|128 samples averaged - signed int16|256 samples averaged - signed int16|-----|4 samples summed - unsigned int16|8 samples summed - unsigned int16|16 samples summed - unsigned int16|32 samples summed - unsigned int16|64 samples summed - unsigned int16|128 samples summed - unsigned int16|256 samples summed - unsigned int16|------|2 samples summed - signed int16|4 samples summed - signed int16|8 samples summed - signed int16|16 samples summed - signed int16|32 samples summed - signed int16|64 samples summed - signed int16|128 samples summed - signed int16|256 samples summed - signed int16),popup(Not used|unsigned int16 |signed int16|---Burst Sample with internal Digital filter---|2 samples averaged - unsigned int16|4 samples averaged - unsigned int16|8 samples averaged - unsigned int16|16 samples averaged - unsigned int16|32 samples averaged - unsigned int16|64 samples averaged - unsigned int16|128 samples averaged - unsigned int16|256 samples averaged - unsigned int16|----|2 samples averaged - signed int16|4 samples averaged - signed int16|8 samples averaged - signed int16|16 samples averaged - signed int16|32 samples averaged - signed int16|64 samples averaged - signed int16|128 samples averaged - signed int16|256 samples averaged - signed int16|-----|4 samples summed - unsigned int16|8 samples summed - unsigned int16|16 samples summed - unsigned int16|32 samples summed - unsigned int16|64 samples summed - unsigned int16|128 samples summed - unsigned int16|256 samples summed - unsigned int16|------|2 samples summed - signed int16|4 samples summed - signed int16|8 samples summed - signed int16|16 samples summed - signed int16|32 samples summed - signed int16|64 samples summed - signed int16|128 samples summed - signed int16|256 samples summed - signed int16),popup(Not used|unsigned int16),popup(Not used|unsigned int16),edit
      mask CallbackString: ||||MCHP_ADC_HighSpeed_SAR_dsPIC_Callback(gcbh,'DialogUpdate');||||||||||||||||MCHP_ADC_HighSpeed_SAR_dsPIC_Callback(gcbh,'DialogUpdate');|||||MCHP_ADC_HighSpeed_SAR_dsPIC_Callback(gcbh,'DialogUpdate');||||||MCHP_ADC_HighSpeed_SAR_dsPIC_Callback(gcbh,'DialogUpdate');|||||MCHP_ADC_HighSpeed_SAR_dsPIC_Callback(gcbh,'DialogUpdate');||||||MCHP_ADC_HighSpeed_SAR_dsPIC_Callback(gcbh,'DialogUpdate');|||||MCHP_ADC_HighSpeed_SAR_dsPIC_Callback(gcbh,'DialogUpdate');||||||MCHP_ADC_HighSpeed_SAR_dsPIC_Callback(gcbh,'DialogUpdate');|||||MCHP_ADC_HighSpeed_SAR_dsPIC_Callback(gcbh,'DialogUpdate');||||||MCHP_ADC_HighSpeed_SAR_dsPIC_Callback(gcbh,'DialogUpdate');|||||MCHP_ADC_HighSpeed_SAR_dsPIC_Callback(gcbh,'DialogUpdate');||||||MCHP_ADC_HighSpeed_SAR_dsPIC_Callback(gcbh,'DialogUpdate');|||||MCHP_ADC_HighSpeed_SAR_dsPIC_Callback(gcbh,'DialogUpdate');||||||MCHP_ADC_HighSpeed_SAR_dsPIC_Callback(gcbh,'DialogUpdate');|||||MCHP_ADC_HighSpeed_SAR_dsPIC_Callback(gcbh,'DialogUpdate');||||||||||||||||||||||||||||||||||||||||||
      mask TabNameString: ADC main,ADC main,ADC main,ADC main,ADC main,ADC main,ADC main,ADC main,ADC main,ADC main,ADC main,ADC main,ADC main,ADC main,ADC main,ADC main,ADC main,ADC main,ADC main,ADC main,ADC0,ADC0,ADC0,ADC0,ADC0,ADC0,ADC0,ADC0,ADC0,ADC0,ADC0,ADC1,ADC1,ADC1,ADC1,ADC1,ADC1,ADC1,ADC1,ADC1,ADC1,ADC1,ADC2,ADC2,ADC2,ADC2,ADC2,ADC2,ADC2,ADC2,ADC2,ADC2,ADC2,ADC3,ADC3,ADC3,ADC3,ADC3,ADC3,ADC3,ADC3,ADC3,ADC3,ADC3,ADC4,ADC4,ADC4,ADC4,ADC4,ADC4,ADC4,ADC4,ADC4,ADC4,ADC4,ADC5,ADC5,ADC5,ADC5,ADC5,ADC5,ADC5,ADC5,ADC5,ADC5,ADC5,ADC6,ADC6,ADC6,ADC6,ADC6,ADC6,ADC6,ADC6,ADC6,ADC6,ADC6,Shared ADC,Shared ADC,Shared ADC,Shared ADC,Shared ADC,Shared ADC,Shared ADC,Shared ADC,Shared ADC,Shared ADC,Shared ADC,Shared ADC,Shared ADC,Shared ADC,Shared ADC,Shared ADC,Shared ADC,Shared ADC,Shared ADC,Shared ADC,Shared ADC,Shared ADC,Shared ADC,Shared ADC,Shared ADC,Shared ADC,Shared ADC,Shared ADC,Shared ADC,Shared ADC,Shared ADC,Shared ADC,Shared ADC,Shared ADC,Shared ADC,Shared ADC,Shared ADC
      mask Display:
      | fprintf('ADC HS SAR\ndsPIC');
      | port_label('output',1,'AN0');
  Analog Comparator Controller (ACC) SAMx : S-Function  InitFcn=MCHP_ACC_SAMx_Callback(gcbh,'InitFcn');  FunctionName=MCHP_ACC_SAMx  Parameters=MCHP_ACC_SAMx_Callback(gcbh,'S_INPUT'),MCHP_ACC_SAMx_Callback(gcbh,'S_OUTPUT'),MCHP_ACC_SAMx_Callback(gcbh,'S_INPUT_Size'),MCHP_ACC_SAMx_Callback(gcbh,'S_OUTPUT_Size'),MCHP_ACC_SAMx_Callback(gcbh,'S_ListCustomDatatype'),SampleTime,0  EnableBusSupport=off  mask(Analog Comparator  (ACC) - SAMx){SELPLUS=Dynamic Options, SELPLUS_TXT=Dynamic Options, SELMINUS=Dynamic Options, SELMINUS_TXT=Dynamic Options, DACC_INITIAL_OUTPUT=1.2, EDGETYP=Rising, INV=off, HYST=Disabled, CE=Disabled, FAULT=Disabled, SampleTime=0.001, S_INPUT=[], S_INPUT_Size=[], S_OUTPUT=[], S_OUTPUT_Size=[], S_ListCustomDatatype=[], MCHP_PORT={TC3}{TIOA9}3:0:P128;, MCHP_MASTERLINK=aaARM_MODEL/Microchip Master, BlockOutput_COMPARATOR_OUTPUT=is not a block output, BlockOutput_COMPARATOR_EDGE_OUTPUT=is not a block output, BlockInput_DACC_INPUT=is not a block input, DACC_SAT=on}
      mask prompts: SELPLUS "Comparator Input: Vin+"; SELPLUS_TXT "Comparator Input: Vin+"; SELMINUS "Comparator Input: Vin-"; SELMINUS_TXT "Comparator Input: Vin-"; DACC_INITIAL_OUTPUT "DAC Initial Output [0V - 3.3V]"; EDGETYP "Comparator Output Edge Type"; INV "Invert Comparator Output"; HYST "Hysteresis"; CE "Comparator Interrupt"; FAULT "PWM Fault Generation"; SampleTime "Sample Time"; BlockOutput_COMPARATOR_OUTPUT "Comparator Output"; BlockOutput_COMPARATOR_EDGE_OUTPUT "Comparator Output Change Detection"; BlockInput_DACC_INPUT "DACC Output Voltage for Vin- Comparator Input"; DACC_SAT "Enable saturation code generation for DACC Input"
      mask help:
      | Tips:
      | Comparator Output Change Detection indicates if a selected edge on analog comparator output occurred since the last read of ACC.
      | * Hover over block configuration parameters for more details.
      mask init:
      | MCHP_ACC_SAMx_Callback(gcbh,'INITIALISATION');
      settings: CopyFcn=MCHP_ACC_SAMx_Callback(gcbh,'CopyFcn');  PreSaveFcn=MCHP_Fun.PreSaveFcn_DynamicOptions(gcbh);  OpenFcn=MCHP_ACC_SAMx_Callback(gcbh,'OPEN');
      mask StyleString: popup(Dynamic Options),edit,popup(Dynamic Options),edit,edit,popup(Rising|Falling|Any),checkbox,popup(Disabled|25 mV|45 mV),popup(Disabled|Enabled (defined by Edge Type)),popup(Disabled|Defined by Edge Type|Defined by Comparator Output),edit,edit,edit,edit,edit,edit,edit,edit,popup(is not a block output|is a boolean block output),popup(is not a block output|is a boolean block output),popup(is not a block input|is a 16 bits unsigned block input in the range [0 - 4026] [0v - 3.3v]|is a Floating Point block input within the range [0 - 1] [0v - 3.3v]|is a Floating Point block input with physical scaling in Volts within the range [0v - 3.3v]),checkbox
      mask CallbackString: ||MCHP_ACC_SAMx_Callback(gcbh,'UpdateGUI');|||||||||||||||||||
      mask TabNameString: Main,Main,Main,Main,Main,Main,Main,Main,Main,Main,Main,Main,Main,Main,Main,Main,Main,Main,Block I/O,Block I/O,Block I/O,Block I/O
      mask Display: fprintf('Analog Comparator \n (ACC) SAMx');
  Comparator - OpAmps - Volt Ref : S-Function  FunctionName=MCHP_COMPARATOR1  Parameters=MCHP_COMPARATOR1_callback(gcbh,'S_INPUT'),MCHP_COMPARATOR1_callback(gcbh,'S_OUTPUT'),MCHP_COMPARATOR1_callback(gcbh,'S_INPUT_Size'),MCHP_COMPARATOR1_callback(gcbh,'S_OUTPUT_Size'),[],SampleTime,MCHP_OrderInOut(gcbh)  EnableBusSupport=off  mask(Comparator / Op amp (DS70357 & DS70648)){MCHP_params=s.CVR1OE=0;s.CVR2OE=0;s.VREFSEL=0;s.RLaddle=reshape([1 1],1,2);s.AVdd=reshape({ '3.3','3.3'},1,2);s.AVss=reshape({ '0','0'},1,2);s.CVRSS=reshape([0 0],1,2);s.CON_OPMODE_CPOL=reshape([0 0 0 0 0],1,5);s.OutputPort_COE_RP=reshape({ 'None','None','None','None','None'},1,5);s.InputP_CREF=reshape([0 0 0 0 0],1,5);s.InputN_CCH=reshape([0 0 0 0 0],1,5);s.Trigger_EventInterrupt_EVPOL=reshape([0 0 0 0 0],1,5);s.BlockOutputEvent=reshape([0 0 0 0 0],1,5);s.BlockOutputState=reshape([0 0 0 0 0],1,5);s.IntPriority=5;s.FilterFreq=reshape([1e+010 1e+010 1e+010 1e+010 1e+010],1,5);s.Blanking=reshape([1 1 1 1 1],1,5);s.BlankingSignal=reshape({ ' - ',' - ',' - ',' - ',' - ',' - ',' - ',' - ',' - ',' - ',' - ',' - ',' - ',' - ',' - '},3,5);s.BlankingTruthTable=reshape([-1 -1 -1 -1 -1 -1 -1 -1 -1 -1 -1 -1 -1 -1 -1 -1 -1 -1 -1 -1 -1 -1 -1 -1 -1 -1 -1 -1 -1 -1 -1 -1 -1 -1 -1 -1 -1 -1 -1 -1 -1 -1 -1 -1 -1 -1 -1 -1 -1 -1 -1 -1 -1 -1 -1 -1 -1 -1 -1 -1 -1 -1 -1 -1 -1 -1 -1 -1 -1 -1 -1 -1 -1 -1 -1 -1 -1 -1 -1 -1 -1 -1 -1 -1 -1 -1 -1 -1 -1 -1 -1 -1 -1 -1 -1 -1 -1 -1 -1 -1 -1 -1 -1 -1 -1 -1 -1 -1 -1 -1 -1 -1 -1 -1 -1 -1 -1 -1 -1 -1 -1 -1 -1 -1 -1 -1 -1 -1 -1 -1 -1 -1 -1 -1 -1 -1 -1 -1 -1 -1 -1 -1 -1 -1 -1 -1 -1 -1 -1 -1 -1 -1 -1 -1 -1 -1 -1 -1 -1 -1 -1 -1 -1 -1 -1 -1 -1 -1 -1 -1 -1 -1 -1 -1 -1 -1 -1 -1 -1 -1 -1 -1 -1 -1 -1 -1 -1 -1 -1 -1 -1 -1 -1 -1 -1 -1 -1 -1 -1 -1 -1 -1 -1 -1 -1 -1 -1 -1 -1 -1 -1 -1 -1 -1 -1 -1 -1 -1 -1 -1 -1 -1 -1 -1 -1 -1 -1 -1 -1 -1 -1 -1 -1 -1 -1 -1 -1 -1 -1 -1],16 ,3 ,5);, S_INPUT=[5  5], S_OUTPUT=[5], S_INPUT_Size=[2  2], S_OUTPUT_Size=[4], SampleTime=-1, MCHP_MASTERLINK=untitled/Microchip Master, MCHP_PORT=, MCHP_USER_INTERRUPTS=, ORDERING=0}
      mask prompts: SampleTime "Sample Time"; ORDERING "MCHP_OrderInOut"
      mask init:
      | MCHP_COMPARATOR1_callback(gcbh,'INITIALISATION');
      settings: CopyFcn=MCHP_COMPARATOR1_callback(gcbh,'COPY');  DeleteFcn=MCHP_COMPARATOR1_callback(gcbh,'DELETE');  ModelCloseFcn=MCHP_COMPARATOR1_callback(gcbh,'MODELCLOSE');  OpenFcn=MCHP_COMPARATOR1_callback(gcbh,'OPEN');
      mask TabNameString: Function,Function,Function,Function,Function,Function,Function,Pins Configuration,Pins Configuration,Pins Configuration
      mask Display: MCHP_DrawLogo;fprintf(['Comparators\nOp-Amps\nVolt Ref']);
  Digital to Analog Converter (DACC) SAMx : S-Function  InitFcn=MCHP_DACC_SAMx_Callback(gcbh,'InitFcn');  FunctionName=MCHP_DACC_SAMx  Parameters=MCHP_DACC_SAMx_Callback(gcbh,'S_INPUT'),MCHP_DACC_SAMx_Callback(gcbh,'S_OUTPUT'),MCHP_DACC_SAMx_Callback(gcbh,'S_INPUT_Size'),MCHP_DACC_SAMx_Callback(gcbh,'S_OUTPUT_Size'),MCHP_DACC_SAMx_Callback(gcbh,'S_ListCustomDatatype'),SampleTime,0  EnableBusSupport=off  mask(Digital to Analog Converter (DACC) - SAMx){DIFF=Single-Ended Outputs, DAC0_OUTPUT_PIN=Dynamic Options, DAC0_OUTPUT_PIN_TXT=Dynamic Options, DAC0_INITIAL_OUTPUT=1.2, DAC1_OUTPUT_PIN=Dynamic Options, DAC1_OUTPUT_PIN_TXT=Dynamic Options, DAC1_INITIAL_OUTPUT=1.2, DAC0_FORCED_OUTPUT_PIN=Dynamic Options, DAC0_FORCED_OUTPUT_PIN_TXT=Dynamic Options, DAC1_FORCED_OUTPUT_PIN=Dynamic Options, DAC1_FORCED_OUTPUT_PIN_TXT=Dynamic Options, DACC_DIFF_INITIAL_OUTPUT=1.2, SampleTime=0.001, S_INPUT=[], S_INPUT_Size=[], S_OUTPUT=[], S_OUTPUT_Size=[], S_ListCustomDatatype=[], MCHP_PORT={TC3}{TIOA9}3:0:P128;, MCHP_MASTERLINK=aaARM_MODEL/Microchip Master, DAC0_INPUT=is a 16 bits unsigned block input, DAC0_INPUT_SAT=on, DAC1_INPUT=is a 16 bits unsigned block input, DAC1_INPUT_SAT=on, DAC_INPUT_DIFF=is a 16 bits unsigned block input, DAC_INPUT_DIFF_SAT=on}
      mask prompts: DIFF "DACC Output Mode"; DAC0_OUTPUT_PIN "DAC0 Output Pin"; DAC0_OUTPUT_PIN_TXT "DAC0 Output Pin_TXT"; DAC0_INITIAL_OUTPUT "DAC0 Initial Output [0V - 3.3V]"; DAC1_OUTPUT_PIN "DAC1 Output Pin"; DAC1_OUTPUT_PIN_TXT "DAC1 Output Pin_TXT"; DAC1_INITIAL_OUTPUT "DAC1 Initial Output [0V - 3.3V]"; DAC0_FORCED_OUTPUT_PIN "DAC0 Output Pin (+)"; DAC0_FORCED_OUTPUT_PIN_TXT "DAC0 Output Pin_TXT"; DAC1_FORCED_OUTPUT_PIN "DAC1 Output Pin (-)"; DAC1_FORCED_OUTPUT_PIN_TXT "DAC1 Output Pin_TXT"; DACC_DIFF_INITIAL_OUTPUT "DACC Initial Output [0V - 3.3V] (Differential Mode)"; SampleTime "Sample Time"; DAC0_INPUT "DAC0 Input"; DAC0_INPUT_SAT "Enable saturation code generation for DAC0 Input"; DAC1_INPUT "DAC1 Input"; DAC1_INPUT_SAT "Enable saturation code generation for DAC1 Input"; DAC_INPUT_DIFF "DAC Input (Differential Mode)"; DAC_INPUT_DIFF_SAT "Enable saturation code generation for DAC Input"
      mask help:
      | Tip:
      | Hover over block configuration parameters for more details.
      mask init:
      | MCHP_DACC_SAMx_Callback(gcbh,'INITIALISATION');
      settings: PreSaveFcn=MCHP_Fun.PreSaveFcn_DynamicOptions(gcbh);  OpenFcn=MCHP_DACC_SAMx_Callback(gcbh,'OPEN');
      mask StyleString: popup(Single-Ended Outputs|Differential Outputs),popup(Dynamic Options),edit,edit,popup(Dynamic Options),edit,edit,popup(Dynamic Options),edit,popup(Dynamic Options),edit,edit,edit,edit,edit,edit,edit,edit,edit,edit,popup(is not a block input|is a 16 bits unsigned block input in the range [0 - 4026] [0v - 3.3v]|is a Floating Point block input within the range [0 - 1] [0v - 3.3v]|is a Floating Point block input with physical scaling in Volts within the range [0v - 3.3v]),checkbox,popup(is not a block input|is a 16 bits unsigned block input in the range [0 - 4026] [0v - 3.3v]|is a Floating Point block input within the range [0 - 1] [0v - 3.3v]|is a Floating Point block input with physical scaling in Volts within the range [0v - 3.3v]),checkbox,popup(is not a block input|is a 16 bits unsigned block input in the range [0 - 4026] [0v - 3.3v]|is a Floating Point block input within the range [0 - 1] [0v - 3.3v]|is a Floating Point block input with physical scaling in Volts within the range [0v - 3.3v]),checkbox
      mask CallbackString: MCHP_DACC_SAMx_Callback(gcbh,'UpdateGUI');|MCHP_DACC_SAMx_Callback(gcbh,'UpdateGUI');|||MCHP_DACC_SAMx_Callback(gcbh,'UpdateGUI');|||||||||||||||||||||
      mask TabNameString: Main,Main,Main,Main,Main,Main,Main,Main,Main,Main,Main,Main,Main,Main,Main,Main,Main,Main,Main,Main,Block I/O,Block I/O,Block I/O,Block I/O,Block I/O,Block I/O
      mask Display: fprintf('Digital-to-Analog Converter (DACC) SAMx');
  High-Speed Analog Comparator : S-Function  InitFcn=MCHP_HighSpeed_AnalogComparator_Callback(gcbh,'InitFcn');  FunctionName=MCHP_HighSpeed_AnalogComparator  Parameters=MCHP_ADC_HighSpeed_SAR_dsPIC_Callback(gcbh,'S_INPUT'),MCHP_ADC_HighSpeed_SAR_dsPIC_Callback(gcbh,'S_OUTPUT'),MCHP_ADC_HighSpeed_SAR_dsPIC_Callback(gcbh,'S_INPUT_Size'),MCHP_ADC_HighSpeed_SAR_dsPIC_Callback(gcbh,'S_OUTPUT_Size'),MCHP_ADC_HighSpeed_SAR_dsPIC_Callback(gcbh,'S_ListCustomDatatype'),SampleTime,0  EnableBusSupport=off  mask(High-Speed Analog Comparator for dSPIC EP GS){Fuse_FDEVOPT_DBCC=off, SampleTime=-1, S_INPUT=[], S_INPUT_Size=[], S_OUTPUT=[5  5], S_OUTPUT_Size=[1  1], S_ListCustomDatatype=S.S_ListCustomDatatype={};, MCHP_USER_INTERRUPTS={AC1}{CMP1}{Analog Comparator 1}{VectorName(CMP1Interrupt) Priority(-1) };, MCHP_PORT=, MCHP_MASTERLINK=Dvpt_33EP64GS504_PGA_ExportForLib/Microchip Master, MCHP_CRC=2217510, Comparator_en1=on, Comparator1_pin=Dynamic Options, Comparator1_pin_TXT=internal signal : PGA1, ExtRef_Range1_pin=Dynamic Options, ExtRef_Range1_pin_TXT=AVdd, ExtRef_Volt1=3.3, CMREF1=2.2, CMREF_Input1=is not modified at run time, HYSSEL_HYSPOL1=45 mV on rising edge, FLTREN1=on, COMP1=is active high, DACOE1=off, StateOut1=on, Comparator_en2=off, Comparator2_pin=Dynamic Options, Comparator2_pin_TXT=CMP2A / A2 / Pin[23], ExtRef_Range2_pin=Dynamic Options, ExtRef_Range2_pin_TXT=AVdd, ExtRef_Volt2=3.3, CMREF2=2.2, CMREF_Input2=is not modified at run time, HYSSEL_HYSPOL2=45 mV on rising edge, FLTREN2=on, COMP2=is active high, DACOE2=off, StateOut2=on, Comparator_en3=off, Comparator3_pin=Dynamic Options, Comparator3_pin_TXT=CMP3A / B9 / Pin[25], ExtRef_Range3_pin=Dynamic Options, ExtRef_Range3_pin_TXT=EXTREF1 / C2 / Pin[36], ExtRef_Volt3=3.3, CMREF3=2.2, CMREF_Input3=is not modified at run time, HYSSEL_HYSPOL3=45 mV on rising edge, FLTREN3=on, COMP3=is active high, DACOE3=off, StateOut3=on, Comparator_en4=off, Comparator4_pin=Dynamic Options, Comparator4_pin_TXT=CMP4A / B1 / Pin[32], ExtRef_Range4_pin=Dynamic Options, ExtRef_Range4_pin_TXT=EXTREF2 / C10 / Pin[28], ExtRef_Volt4=3.3, CMREF4=2.2, CMREF_Input4=is a block input value within [0 4095] coding for 0V to ref Volt, HYSSEL_HYSPOL4=45 mV on rising edge, FLTREN4=on, COMP4=is active high, DACOE4=off, StateOut4=on}
      mask prompts: Fuse_FDEVOPT_DBCC "Connect DACOUT1 with DACOUT2 (set in Master Block)"; SampleTime "Block output sample time"; Comparator_en1 "Enable High-Speed Comparator 1"; Comparator1_pin "Comparator input"; Comparator1_pin_TXT "Comparator input"; ExtRef_Range1_pin "Comparator Reference Voltage"; ExtRef_Range1_pin_TXT "Comparator Reference Voltage"; ExtRef_Volt1 "Reference Voltage input (V)"; CMREF1 "Initial comparator threshold set to (V)"; CMREF_Input1 "Comparator threshold"; HYSSEL_HYSPOL1 "Hysteresis"; FLTREN1 "Digital Filter Comparator Output (Fc = 320000kHz)"; COMP1 "Comparator Output Polarity"; DACOE1 "Connect comparator threshold to DACOUT1 Pin (B3 / Pin[34] )"; StateOut1 "Comparator State (including Polarity setting) is a block output"; Comparator_en2 "Enable High-Speed Comparator 1"; Comparator2_pin "Comparator input"; Comparator2_pin_TXT "Comparator input"; ExtRef_Range2_pin "Comparator Reference Voltage"; ExtRef_Range2_pin_TXT "Comparator Reference Voltage"; ExtRef_Volt2 "Reference Voltage input (V)"; CMREF2 "Initial comparator threshold set to (V)"; CMREF_Input2 "Comparator threshold"; HYSSEL_HYSPOL2 "Hysteresis"; FLTREN2 "Digital Filter Comparator Output (Fc = 320000kHz)"; COMP2 "Comparator Output Polarity"; DACOE2 "Connect comparator threshold to DACOUT2 (Internal signal only)"; StateOut2 "Comparator State (including Polarity setting) is a block output"; Comparator_en3 "Enable High-Speed Comparator 1"; Comparator3_pin "Comparator input"; Comparator3_pin_TXT "Comparator input"; ExtRef_Range3_pin "Comparator Reference Voltage"; ExtRef_Range3_pin_TXT "Comparator Reference Voltage"; ExtRef_Volt3 "Reference Voltage input (V)"; CMREF3 "Initial comparator threshold set to (V)"; CMREF_Input3 "Comparator threshold"; HYSSEL_HYSPOL3 "Hysteresis"; FLTREN3 "Digital Filter Comparator Output (Fc = 320000kHz)"; COMP3 "Comparator Output Polarity"; DACOE3 "Connect comparator threshold to DACOUT1 Pin (B3 / Pin[34] )"; StateOut3 "Comparator State (including Polarity setting) is a block output"; Comparator_en4 "Enable High-Speed Comparator 1"; Comparator4_pin "Comparator input"; Comparator4_pin_TXT "Comparator input"; ExtRef_Range4_pin "Comparator Reference Voltage"; ExtRef_Range4_pin_TXT "Comparator Reference Voltage"; ExtRef_Volt4 "Reference Voltage input (V)"; CMREF4 "Initial comparator threshold set to (V)"; CMREF_Input4 "Comparator threshold"; HYSSEL_HYSPOL4 "Hysteresis"; FLTREN4 "Digital Filter Comparator Output (Fc = 320000kHz)"; COMP4 "Comparator Output Polarity"; DACOE4 "Connect comparator threshold to DACOUT2 (Internal signal only)"; StateOut4 "Comparator State (including Polarity setting) is a block output"
      mask help:
      | Compare input signal or input from PGA peripheral to a threshold.
      | The PGA block creates users interrupts allowing to trig asynchronously subsystem with the Interruption block available.
      mask init:
      | MCHP_HighSpeed_AnalogComparator_Callback(gcbh,'INITIALISATION');
      settings: CopyFcn=MCHP_HighSpeed_AnalogComparator_Callback(gcbh,'CopyFcn');  PreSaveFcn=MCHP_Fun.PreSaveFcn_DynamicOptions(gcbh);  OpenFcn=MCHP_HighSpeed_AnalogComparator_Callback(gcbh,'OPEN');
      mask StyleString: checkbox,edit,edit,edit,edit,edit,edit,edit,edit,edit,edit,checkbox,popup(Dynamic Options),edit,popup(Dynamic Options),edit,edit,edit,popup(is not modified at run time|is a block input value within [0 4095] coding for 0V to ref Volt),popup(No Hysteresis|15 mV on rising edge|30 mV on rising edge|45 mV on rising edge|---|15 mV on falling edge|30 mV on falling edge|45 mV on falling edge),checkbox,popup(is active high|is active low),checkbox,checkbox,checkbox,popup(Dynamic Options),edit,popup(Dynamic Options),edit,edit,edit,popup(is not modified at run time|is a block input value within [0 4095] coding for 0V to ref Volt),popup(No Hysteresis|15 mV on rising edge|30 mV on rising edge|45 mV on rising edge|---|15 mV on falling edge|30 mV on falling edge|45 mV on falling edge),checkbox,popup(is active high|is active low),checkbox,checkbox,checkbox,popup(Dynamic Options),edit,popup(Dynamic Options),edit,edit,edit,popup(is not modified at run time|is a block input value within [0 4095] coding for 0V to ref Volt),popup(No Hysteresis|15 mV on rising edge|30 mV on rising edge|45 mV on rising edge|---|15 mV on falling edge|30 mV on falling edge|45 mV on falling edge),checkbox,popup(is active high|is active low),checkbox,checkbox,checkbox,popup(Dynamic Options),edit,popup(Dynamic Options),edit,edit,edit,popup(is not modified at run time|is a block input value within [0 4095] coding for 0V to ref Volt),popup(No Hysteresis|15 mV on rising edge|30 mV on rising edge|45 mV on rising edge|---|15 mV on falling edge|30 mV on falling edge|45 mV on falling edge),checkbox,popup(is active high|is active low),checkbox,checkbox
      mask CallbackString: |||||||||||MCHP_HighSpeed_AnalogComparator_Callback(gcbh,'Comparator_en1');|||||||||||||MCHP_HighSpeed_AnalogComparator_Callback(gcbh,'Comparator_en2');|||||||||||||MCHP_HighSpeed_AnalogComparator_Callback(gcbh,'Comparator_en3');|||||||||||||MCHP_HighSpeed_AnalogComparator_Callback(gcbh,'Comparator_en4');||||||||||||
      mask TabNameString: General,General,General,General,General,General,General,General,General,General,General,CMP1,CMP1,CMP1,CMP1,CMP1,CMP1,CMP1,CMP1,CMP1,CMP1,CMP1,CMP1,CMP1,CMP2,CMP2,CMP2,CMP2,CMP2,CMP2,CMP2,CMP2,CMP2,CMP2,CMP2,CMP2,CMP2,CMP3,CMP3,CMP3,CMP3,CMP3,CMP3,CMP3,CMP3,CMP3,CMP3,CMP3,CMP3,CMP3,CMP4,CMP4,CMP4,CMP4,CMP4,CMP4,CMP4,CMP4,CMP4,CMP4,CMP4,CMP4,CMP4
      mask Display:
      | fprintf('HighSpeed_AnalogComparator');
      | port_label('output',1,'CMP1');
  Op-Amp : S-Function  Priority=-2000  InitFcn=MCHP_OP_AMP_Callback(gcbh,'InitFcn');  FunctionName=MCHP_OP_AMP  Parameters=[],[],[],[],[],-1,0  EnableBusSupport=off  mask(Configure on chip Op AMP){OpAmp1=Enabled with positive and negative inputs, OpAmp2=Disabled, OpAmp3=Disabled, S_INPUT=[-1], S_INPUT_Size=[3], S_OUTPUT=[], S_OUTPUT_Size=[], S_ListCustomDatatype=S.S_ListCustomDatatype={};, MCHP_USER_INTERRUPTS=0, MCHP_PORT={OA1 Output}{OA1out}14:2:A0;{OA1 IN+}{OA1in+}14:2:A2;{OA1 IN-}{OA1in-}14:2:A1;, MCHP_MASTERLINK=dsPIC33CK_OpAmp_R2014b/Microchip Master, MCHP_CRC=406585, INFO=}
      mask prompts: OpAmp1 "Op-Amp1 In+/In-/Out => A2(AN9) / A1 / A0(AN0)"; OpAmp2 "Op-Amp2 In+/In-/Out => B4 / B3(AN8) / B2(AN1)"; OpAmp3 "Op-Amp3 In+/In-/Out => C2(AN14) / C1(AN13) / A4(AN4)"; INFO "Infos"
      mask help: Configure the Op Amp available on the dsPIC CK family
      mask init:
      | MCHP_OP_AMP_Callback(gcbh,'INITIALISATION');
      settings: CopyFcn=MCHP_OP_AMP_Callback(gcbh,'CopyFcn');  PreSaveFcn=MCHP_Fun.PreSaveFcn_DynamicOptions(gcbh);  OpenFcn=MCHP_OP_AMP_Callback(gcbh,'OPEN');
      mask StyleString: popup(Disabled|Enabled with negative input internally set to 0|Enabled with positive and negative inputs),popup(Disabled|Enabled with negative input internally set to 0|Enabled with positive and negative inputs),popup(Disabled|Enabled with negative input internally set to 0|Enabled with positive and negative inputs),edit,edit,edit,edit,edit,edit,edit,edit,edit,edit
      mask TabNameString: Initialisation,Initialisation,Initialisation,Initialisation,Initialisation,Initialisation,Initialisation,Initialisation,Initialisation,Initialisation,Initialisation,Initialisation,Initialisation
      mask Display: fprintf('Op-Amp');
  PGA - Programmable Gain Amplifier : S-Function  InitFcn=MCHP_PGA_Callback(gcbh,'InitFcn');  FunctionName=MCHP_PGA  Parameters=MCHP_ADC_HighSpeed_SAR_dsPIC_Callback(gcbh,'S_INPUT'),MCHP_ADC_HighSpeed_SAR_dsPIC_Callback(gcbh,'S_OUTPUT'),MCHP_ADC_HighSpeed_SAR_dsPIC_Callback(gcbh,'S_INPUT_Size'),MCHP_ADC_HighSpeed_SAR_dsPIC_Callback(gcbh,'S_OUTPUT_Size'),MCHP_ADC_HighSpeed_SAR_dsPIC_Callback(gcbh,'S_ListCustomDatatype'),SampleTime,0  EnableBusSupport=off  mask(Programmable Gain Amplifier for dsPIC EP GS ){Fuse_FDEVOPT_DBCC=off, PGA1Gain=Gain of 4x, PGA1Gain_BlockInput=off, PGA1P_pin=Dynamic Options, PGA1P_pin_TXT=PGA1P1 / A0 / Pin[21], PGA1N_pin=Dynamic Options, PGA1N_pin_TXT=Ground (Single-Ended mode), PGA1Output=on, PGA2Gain=Disabled, PGA2Gain_BlockInput=off, PGA2P_pin=Dynamic Options, PGA2P_pin_TXT=PGA2P2 / A2 / Pin[23], PGA2N_pin=Dynamic Options, PGA2N_pin_TXT=PGA2N2 / B5 / Pin[43], PGA2Output=off, SampleTime=.001, S_INPUT=[], S_INPUT_Size=[], S_OUTPUT=[5  5], S_OUTPUT_Size=[1  1], S_ListCustomDatatype=S.S_ListCustomDatatype={};, MCHP_USER_INTERRUPTS={ADCAN0}{ADCBUF0}{ADC Data 0 Ready}{VectorName(ADCAN0Interrupt) Priority(-1) RegisterReadClear(ADCBUF0)Config_BitSet(ADIELbits.IE0) };, MCHP_PORT={AMP PGA1OUT}{PGA1OUT}14:2:B3;{AMP PGA1 (+)}{PGA1(+)}14:2:A0;, MCHP_MASTERLINK=Dvpt_33EP64GS504_PGA_ExportForLib/Microchip Master, MCHP_CRC=869832}
      mask prompts: Fuse_FDEVOPT_DBCC "Connect DACOUT1 with DACOUT2 (set in Master Block)"; PGA1Gain "----- Gain 1 ----- (PGA1)"; PGA1Gain_BlockInput "Modify Gain1 at run time (Gain is 2^input ; input in [2 6])"; PGA1P_pin "PGA1 Positive Input"; PGA1P_pin_TXT "PGA1 Positive Input"; PGA1N_pin "PGA1 Negative Input"; PGA1N_pin_TXT "PGA1 Negative Input"; PGA1Output "Connect Gain output to DACOUT1 Port (B3 / Pin[34] )"; PGA2Gain "----- Gain 2 ----- (PGA2)"; PGA2Gain_BlockInput "Modify Gain2 at run time (Gain is 2^input ; input in [2 6])"; PGA2P_pin "PGA2 Positive Input"; PGA2P_pin_TXT "PGA2 Positive Input"; PGA2N_pin "PGA2 Negative Input"; PGA2N_pin_TXT "PGA2 Negative Input"; PGA2Output "Connect Gain output to DACOUT2 (Internal signal only)"; SampleTime "Block output sample time"
      mask help:
      | Op-Amp based non inverting amplifier with user programmable gains.
      | Gain setting can be 4x, 8x, 16x, 32x or 64x.
      | Output of PGA can be internally connected to ADC input or to high-speed comparator module.
      | Output of PGA can also be available on PGAxOUT pin.
      mask init:
      | MCHP_PGA_Callback(gcbh,'INITIALISATION');
      settings: CopyFcn=MCHP_PGA_Callback(gcbh,'CopyFcn');  PreSaveFcn=MCHP_Fun.PreSaveFcn_DynamicOptions(gcbh);  OpenFcn=MCHP_PGA_Callback(gcbh,'OPEN');
      mask StyleString: checkbox,popup(Disabled|Gain of 4x|Gain of 8x|Gain of 16x|Gain of 32x|Gain of 64x),checkbox,popup(Dynamic Options),edit,popup(Dynamic Options),edit,checkbox,popup(Disabled|Gain of 4x|Gain of 8x|Gain of 16x|Gain of 32x|Gain of 64x),checkbox,popup(Dynamic Options),edit,popup(Dynamic Options),edit,checkbox,edit,edit,edit,edit,edit,edit,edit,edit,edit,edit
      mask CallbackString: |MCHP_PGA_Callback(gcbh,'PGA1Gain');|MCHP_PGA_Callback(gcbh,'PGA1Gain_BlockInput');||||||MCHP_PGA_Callback(gcbh,'PGA2Gain');|MCHP_PGA_Callback(gcbh,'PGA2Gain_BlockInput');|||||||||||||||
      mask TabNameString: PGA1 and PGA2,PGA1 and PGA2,PGA1 and PGA2,PGA1 and PGA2,PGA1 and PGA2,PGA1 and PGA2,PGA1 and PGA2,PGA1 and PGA2,PGA1 and PGA2,PGA1 and PGA2,PGA1 and PGA2,PGA1 and PGA2,PGA1 and PGA2,PGA1 and PGA2,PGA1 and PGA2,PGA1 and PGA2,PGA1 and PGA2,PGA1 and PGA2,PGA1 and PGA2,PGA1 and PGA2,PGA1 and PGA2,PGA1 and PGA2,PGA1 and PGA2,PGA1 and PGA2,PGA1 and PGA2
      mask Display: fprintf('PGA');
